simulink model "MPCControlOffshore"  (R2023a)
settings: Solver=VariableStepAuto  StartTime=0.0  StopTime=10.0  RelTol=1e-3
undefined symbols (not defined in the file): A, Amplitude, C1, C2, C3, C4, C_p, L1, L2, L3, Resistance, Ts_Power, v
libraries: spsSeriesRLCBranchLib x11, spsVoltageMeasurementLib x6, spsCurrentMeasurementLib x4, spsDiodeLib x4, spsMosfetLib x1, spsPVArrayLib x1, spsControlledVoltageSourceLib x1, simulink x1, spsDCVoltageSourceLib x1, spspowerguiLib x1
settings Model: Creator=ovais  LastModifiedBy=ovais

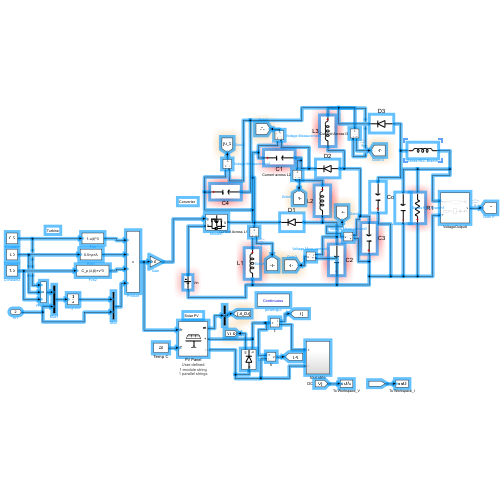
[thumbnail: Simulink's stored preview of the top-level diagram]
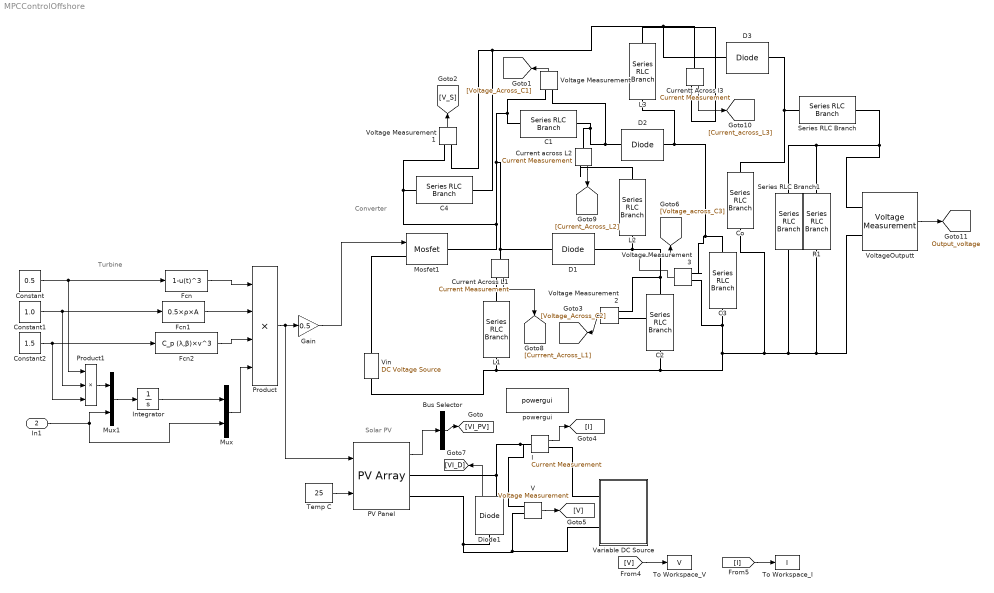
== system MPCControlOffshore ==
  note: Turbine
  note: Solar PV
  note: Converter
  In1 : Inport  Port=2
  Bus Selector : BusSelector  OutputSignals=V_PV,I_PV  OutputAsBus=on
  C1 : spsSeriesRLCBranchLib/Series RLC Branch  LConnTagsString=__new0  RConnTagsString=__new0  BranchType=C  Resistance=1  Inductance=1e-3  SetiL0=off  InitialCurrent=0  Capacitance=C1  Setx0=off  InitialVoltage=0  Measurements=None
  C2 : spsSeriesRLCBranchLib/Series RLC Branch  LConnTagsString=__new0  RConnTagsString=__new0  BranchType=C  Resistance=1  Inductance=1e-3  SetiL0=off  InitialCurrent=0  Capacitance=C2  Setx0=off  InitialVoltage=0  Measurements=None
  C3 : spsSeriesRLCBranchLib/Series RLC Branch  LConnTagsString=__new0  RConnTagsString=__new0  BranchType=C  Resistance=1  Inductance=1e-3  SetiL0=off  InitialCurrent=0  Capacitance=C3  Setx0=off  InitialVoltage=0  Measurements=None
  C4 : spsSeriesRLCBranchLib/Series RLC Branch  LConnTagsString=__new0  RConnTagsString=__new0  BranchType=C  Resistance=1  Inductance=1e-3  SetiL0=off  InitialCurrent=0  Capacitance=C4  Setx0=off  InitialVoltage=0  Measurements=None
  Co : spsSeriesRLCBranchLib/Series RLC Branch  LConnTagsString=__new0  RConnTagsString=__new0  BranchType=C  Resistance=1  Inductance=1e-3  SetiL0=off  InitialCurrent=0  Capacitance=800e-6  Setx0=off  InitialVoltage=0  Measurements=None
  Constant : Constant  Value=0.5
  Constant1 : Constant  Value=1.0
  Constant2 : Constant  Value=1.5
  Current Across L1 : spsCurrentMeasurementLib/Current Measurement  PhasorSimulation=off  OutputType=Complex  PSBequivalent=0
  Current across L2 : spsCurrentMeasurementLib/Current Measurement  PhasorSimulation=off  OutputType=Complex  PSBequivalent=0
  Currentt Across l3 : spsCurrentMeasurementLib/Current Measurement  PhasorSimulation=off  OutputType=Complex  PSBequivalent=0
  D1 : spsDiodeLib/Diode  Ron=1e-6  Lon=0  Vf=0.8  IC=0  UseSnubber=0  Rs=500  Cs=250e-9  Measurements=off
  D2 : spsDiodeLib/Diode  Ron=1e-6  Lon=0  Vf=0.8  IC=0  UseSnubber=0  Rs=500  Cs=250e-9  Measurements=off
  D3 : spsDiodeLib/Diode  Ron=1e-6  Lon=0  Vf=0.8  IC=0  UseSnubber=0  Rs=500  Cs=250e-9  Measurements=off
  Diode1 : spsDiodeLib/Diode  Ron=0.001  Lon=0  Vf=0.7  IC=0  UseSnubber=off  Rs=1e5*inf  Cs=inf  Measurements=on
  Fcn : Fcn  Expr=1-u(t)^3
  Fcn1 : Fcn  Expr=0.5×ρ×A
  Fcn2 : Fcn  Expr=C_p (λ,β)×v^3
  Gain : Gain  Gain=0.5
  I : spsCurrentMeasurementLib/Current Measurement  PhasorSimulation=off  OutputType=Complex  PSBequivalent=0
  Integrator : Integrator
  L1 : spsSeriesRLCBranchLib/Series RLC Branch  LConnTagsString=__new0  RConnTagsString=__new0  BranchType=L  Resistance=1  Inductance=L1  SetiL0=off  InitialCurrent=0  Capacitance=1e-6  Setx0=off  InitialVoltage=0  Measurements=None
  L2 : spsSeriesRLCBranchLib/Series RLC Branch  LConnTagsString=__new0  RConnTagsString=__new0  BranchType=L  Resistance=1  Inductance=L2  SetiL0=off  InitialCurrent=0  Capacitance=1e-6  Setx0=off  InitialVoltage=0  Measurements=None
  L3 : spsSeriesRLCBranchLib/Series RLC Branch  LConnTagsString=__new0  RConnTagsString=__new0  BranchType=L  Resistance=1  Inductance=L3  SetiL0=off  InitialCurrent=0  Capacitance=1e-6  Setx0=off  InitialVoltage=0  Measurements=None
  Mosfet1 : spsMosfetLib/Mosfet  Ron=0.1e-6  Lon=0  Rd=0.1e-6  Vfd=0  IC=0  Rs=1e5  Cs=inf  Measurements=off
  Mux : Mux  Inputs=2
  Mux1 : Mux  Inputs=2
  PV Panel : spsPVArrayLib/PV Array  Npar=1  Nser=1  PlotType=one module @ 25 deg.C & specified irradiances  S_vec=1000  Temp_C_vec="[ 45 25  ]"  ModuleName=User-defined  PlotWhenSelected=off  Pm=59.85  Ncell=36  Voc=21.1  Isc=3.8  Vm=17.1  Im=3.5  beta_Voc_pc=-0.38  alpha_Isc_pc=0.065  beta_Voc=-0.08018  alpha_Isc=0.00247  IL=3.8128  I0=2.5245e-10  nI=0.97484  Rsh=153.5644  Rs=0.38572  RobustModel=off  RobustCellTemperature=313.3991  BAL=off  Tc=1e-6  Tfilter=0.0001
      settings: AttributesFormatString=|
      | %<ModuleName>
      | %<Nser>-module string
      | %<Npar> parallel strings
  Product : Product  Inputs=4
  Product1 : Product  Inputs=3
  R1 : spsSeriesRLCBranchLib/Series RLC Branch  LConnTagsString=__new0  RConnTagsString=__new0  BranchType=R  Resistance=Resistance  Inductance=1e-3  SetiL0=off  InitialCurrent=0  Capacitance=1e-6  Setx0=off  InitialVoltage=0  Measurements=None
  Series RLC Branch : spsSeriesRLCBranchLib/Series RLC Branch  LConnTagsString=__new0  RConnTagsString=__new0  BranchType=L  Resistance=1  Inductance=100e-9  SetiL0=off  InitialCurrent=0  Capacitance=1e-6  Setx0=off  InitialVoltage=0  Measurements=None
  Series RLC Branch1 : spsSeriesRLCBranchLib/Series RLC Branch  LConnTagsString=__new0  RConnTagsString=__new0  BranchType=C  Resistance=1  Inductance=100e-9  SetiL0=off  InitialCurrent=0  Capacitance=33e-6  Setx0=off  InitialVoltage=0  Measurements=None
  Temp C : Constant  Value=25
  To Workspace_I : ToWorkspace  VariableName=I  SampleTime=1e-3
  To Workspace_V : ToWorkspace  VariableName=V  SampleTime=1e-3
  V : spsVoltageMeasurementLib/Voltage Measurement  PhasorSimulation=off  OutputType=Complex  PSBequivalent=0
  Variable DC Source : Subsystem
  Vin : spsDCVoltageSourceLib/DC Voltage Source  Amplitude=Amplitude  Measurements=None
  Voltage Measurement{,1..3} (4 alike) : spsVoltageMeasurementLib/Voltage Measurement  PhasorSimulation=off  OutputType=Complex  PSBequivalent=0
  VoltageOutputt : spsVoltageMeasurementLib/Voltage Measurement  PhasorSimulation=off  OutputType=Complex  PSBequivalent=0
  powergui : spspowerguiLib/powergui  Priority=1  SimulationMode=Continuous  SampleTime=Ts_Power*0 + 20e-6  frequency=60  Iterations=50  frequencyindice=0  Pbase=100e6  ErrMax=1e-4  UnitsV=kV  UnitsW=MW  buscounter=0  FunctionMessages=off  echomessages=off  EnableUseOfTLC=off  CurrentSourceSwitches=off  DisableSnubberDevices=on  DisableRonSwitches=off  DisableVfSwitches=off  DisplayEquations=off  AutomaticDiscreteSolvers=off  SolverType=Tustin/Backward Euler (TBE)  Interpol=off  ExternalGateDelay=off  methode=off  Ts=0  x0status=blocks  SPID=off  SwTol=0  HookPort=off  NonlinearTolerance=1e-4  nMaxIteration=100  ContinueOnMaxIteration=off  RestoreLinks=warning  ResistiveCurrentMeasurement=off  Frange=[0:2:500]  Ylog=off  Xlog=on  ShowGrid=off  save=off  variable=ZData  structure=0  ZoomFFT=on  StartTime=0.0  cycles=1  DisplayStyle=1  fundamental=60  FreqAxis=off  MaxFrequency=1000  frequencyindicesteady=1  RmsSteady=1  display=off
  tag scope: Output_voltage=global
  wires:
  Product/1 -> PV Panel/1, Gain/1
  Fcn/1 -> Product/1
  Constant/1 -> Product1/1, Fcn/1
  Constant1/1 -> Product1/2, Fcn1/1
  Fcn1/1 -> Product/2
  Constant2/1 -> Product1/3, Fcn2/1
  Fcn2/1 -> Product/3
  Integrator/1 -> Mux/1
  Mux/1 -> Product/4
  In1/1 -> Mux/2, Mux1/2
  Mux1/1 -> Integrator/1
  Product1/1 -> Mux1/1
  Temp C/1 -> PV Panel/2
  I/1 -> [I]
  [I] -> To Workspace_I/1
  PV Panel/1 -> Bus Selector/1
  Bus Selector/1 -> [VI_PV]
  Diode1/1 -> [VI_D]
  V/1 -> [V]
  [V] -> To Workspace_V/1
  Voltage Measurement2/1 -> [Voltage_Across_C2]
  Voltage Measurement3/1 -> [Voltage_across_C3]
  Current across L2/1 -> [Current_Across_L2]
  Voltage Measurement1/1 -> [V_S]
  Current Across L1/1 -> [Currrent_Across_L1]
  Currentt Across l3/1 -> [Current_across_L3]
  Voltage Measurement/1 -> [Voltage_Across_C1]
  VoltageOutputt/1 -> [Output_voltage]
  Gain/1 -> Mosfet1/1
  connections:
  Diode1/RConn1 -- V/LConn1 -- I/LConn1 -- PV Panel/RConn1
  Variable DC Source/LConn2 -- PV Panel/RConn2 -- Diode1/LConn1 -- V/LConn2
  I/RConn1 -- Variable DC Source/LConn1
  R1/RConn1 -- Series RLC Branch/RConn1 -- VoltageOutputt/LConn2 -- Series RLC Branch1/RConn1
  C3/RConn1 -- Voltage Measurement3/LConn2 -- L3/RConn1 -- D2/LConn1
  D1/LConn1 -- L2/RConn1 -- Voltage Measurement2/LConn2 -- C2/RConn1
  Voltage Measurement1/LConn1 -- C4/LConn1 -- Voltage Measurement/LConn1 -- C1/LConn1 -- Current Across L1/LConn1 -- D1/RConn1 -- Mosfet1/RConn1
  Co/LConn1 -- VoltageOutputt/LConn1 -- R1/LConn1 -- Series RLC Branch1/LConn1 -- Voltage Measurement3/LConn1 -- C3/LConn1 -- Voltage Measurement2/LConn1 -- Vin/LConn1 -- L1/RConn1
  C4/RConn1 -- Currentt Across l3/LConn1 -- D3/RConn1 -- Voltage Measurement1/LConn2
  Current across L2/LConn1 -- C1/RConn1 -- Voltage Measurement/LConn2 -- D2/RConn1
  Series RLC Branch/LConn1 -- D3/LConn1 -- Co/RConn1
  Currentt Across l3/RConn1 -- L3/LConn1
  Mosfet1/LConn1 -- Vin/RConn1
  Current across L2/RConn1 -- L2/LConn1
  Current Across L1/RConn1 -- L1/LConn1

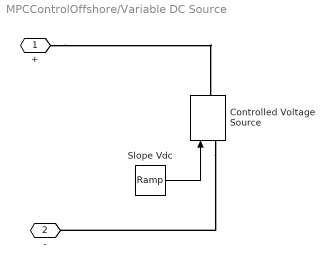
== system MPCControlOffshore/Variable DC Source ==
  Controlled Voltage Source : spsControlledVoltageSourceLib/Controlled Voltage Source  Initialize=on  Source_Type=AC  Amplitude=0  Phase=0  Frequency=0  Measurements=None
  Slope Vdc : simulink/Sources/Ramp  slope=21.1  start=0  InitialOutput=0
  + : PMIOPort  Side=Left
  - : PMIOPort  Port=2  Side=Left
  wires:
  Slope Vdc/1 -> Controlled Voltage Source/1
  connections:
  Controlled Voltage Source/LConn1 -- -/RConn1
  +/RConn1 -- Controlled Voltage Source/RConn1
